simulink model "VL29"  (Simulink 10.1)
settings: Solver=ode3  StartTime=0.0  StopTime=10000.0  FixedStep=Auto  RelTol=1e-3  EnableMultiTasking=on
values from neighbouring files (symbols this model uses):
  In1 = 1    [juece.m]
  In2 = 1    [juece.m]
undefined symbols (not defined in the file): kd1, kd2, ki1, ki2, kp1, kp2
settings Model: Creator=l  LastModifiedBy=97038
settings SolverCC: ShapePreserveControl=EnableAll
settings DataIOCC: LimitDataPoints=on
settings DebuggingCC: UnderspecifiedInitializationDetection=Simplified  MergeDetectMultiDrivingBlocksExec=error  SolverPrmCheckMsg=warning  SFExecutionAtInitializationDiag=warning
settings GRTTargetCC: CombineOutputUpdateFcns=on  GRTInterface=off
settings ConfigComp: CovSFcnEnable=off

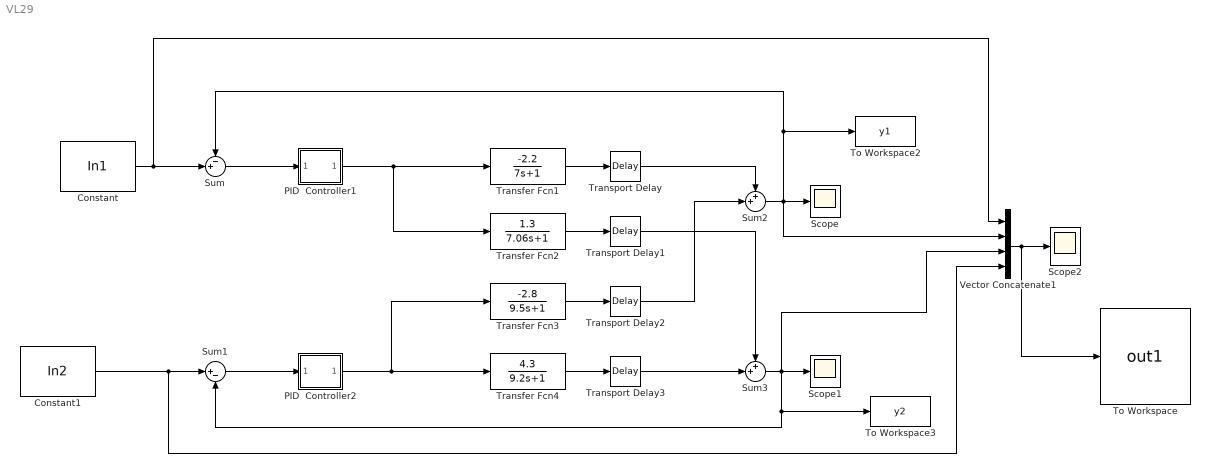
== system VL29 ==
  Constant : Constant  Value=In1
  Constant1 : Constant  Value=In2
  PID  Controller1 : Subsystem  mask(PID Controller){P=kp1, I=ki1, D=kd1}
      mask prompts: P "Proportional:"; I "Integral"; D "Derivative:"
      mask help:
      | Enter expressions for proportional, integral, and derivative terms.
      | P+I/s+Ds
      mask Help: This block implements a PID controller where parameters are entered for the Proportional, Integral and Derivative terms. Unmask this block to see how it works. The derivative term is implemented using a true derivative block.
      mask Display: disp('PID')
  PID  Controller2 : Subsystem  mask(PID Controller){P=kp2, I=ki2, D=kd2}
      mask prompts: P "Proportional:"; I "Integral"; D "Derivative:"
      mask help:
      | Enter expressions for proportional, integral, and derivative terms.
      | P+I/s+Ds
      mask Help: This block implements a PID controller where parameters are entered for the Proportional, Integral and Derivative terms. Unmask this block to see how it works. The derivative term is implemented using a true derivative block.
      mask Display: disp('PID')
  Scope : Scope
  Scope1 : Scope
  Scope2 : Scope
  Sum : Sum  Inputs=-+|  SampleTime=1
  Sum1 : Sum  Inputs=|+-  SampleTime=1
  Sum2 : Sum  Inputs=++|  SampleTime=1
  Sum3 : Sum  Inputs=++|  SampleTime=1
  To Workspace : ToWorkspace  VariableName=out1  SaveFormat=Timeseries  SampleTime=-1
  To Workspace2 : ToWorkspace  VariableName=y1  SampleTime=-1
      settings: Save2DSignal=2-D array (concatenate along first dimension)
  To Workspace3 : ToWorkspace  VariableName=y2  SampleTime=-1
      settings: Save2DSignal=2-D array (concatenate along first dimension)
  Transfer Fcn1 : TransferFcn  Numerator=[-2.2]  Denominator=[7 1]  ContinuousStateAttributes='G11'
  Transfer Fcn2 : TransferFcn  Numerator=[1.3]  Denominator=[7.06 1]  ContinuousStateAttributes='G12'
  Transfer Fcn3 : TransferFcn  Numerator=[-2.8]  Denominator=[9.5 1]
  Transfer Fcn4 : TransferFcn  Numerator=[4.3]  Denominator=[9.2 1]
  Transport Delay : TransportDelay
  Transport Delay1 : TransportDelay  DelayTime=0.3
  Transport Delay2 : TransportDelay  DelayTime=1.8
  Transport Delay3 : TransportDelay  DelayTime=0.35
  Vector Concatenate1 : Concatenate  NumInputs=4
  wires:
  Transfer Fcn1/1 -> Transport Delay/1
  Transfer Fcn2/1 -> Transport Delay1/1
  Transfer Fcn3/1 -> Transport Delay2/1
  Transfer Fcn4/1 -> Transport Delay3/1
  PID  Controller1/1(Out_1) -> Transfer Fcn2/1, Transfer Fcn1/1
  PID  Controller2/1(Out_1) -> Transfer Fcn3/1, Transfer Fcn4/1
  Sum3/1 -> Vector Concatenate1/3, Scope1/1, To Workspace3/1, Sum1/2
  Sum/1 -> PID  Controller1/1(In_1)
  Sum1/1 -> PID  Controller2/1(In_1)
  Constant1/1 -> Vector Concatenate1/4, Sum1/1
  Transport Delay/1 -> Sum2/1
  Transport Delay3/1 -> Sum3/2
  Sum2/1 -> Vector Concatenate1/2, To Workspace2/1, Sum/1, Scope/1
  Vector Concatenate1/1 -> To Workspace/1, Scope2/1
  Transport Delay1/1 -> Sum3/1
  Transport Delay2/1 -> Sum2/2
  Constant/1 -> Vector Concatenate1/1, Sum/2

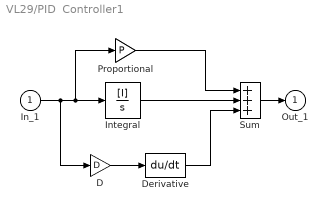
== system VL29/PID  Controller1 ==
  In_1 : Inport
  D : Gain  Gain=D  SaturateOnIntegerOverflow=on  OutDataTypeStr=Inherit: Same as input  ParamDataTypeStr=Inherit: Same as input
  Derivative : Derivative
  Integral : TransferFcn  Numerator=[I]  Denominator=[1 0]
  Proportional : Gain  Gain=P  SaturateOnIntegerOverflow=on  OutDataTypeStr=Inherit: Same as input  ParamDataTypeStr=Inherit: Same as input
  Sum : Sum  Inputs=+++  InputSameDT=on  SaturateOnIntegerOverflow=on  OutDataTypeStr=Inherit: Same as first input
  Out_1 : Outport  InitialOutput=0
  wires:
  D/1 -> Derivative/1
  Sum/1 -> Out_1/1
  In_1/1 -> D/1, Proportional/1, Integral/1
  Derivative/1 -> Sum/3
  Integral/1 -> Sum/2
  Proportional/1 -> Sum/1

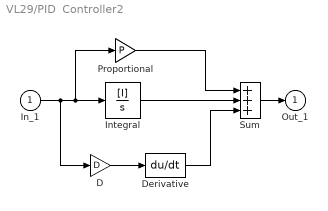
== system VL29/PID  Controller2 ==
  In_1 : Inport
  D : Gain  Gain=D  SaturateOnIntegerOverflow=on  OutDataTypeStr=Inherit: Same as input  ParamDataTypeStr=Inherit: Same as input
  Derivative : Derivative
  Integral : TransferFcn  Numerator=[I]  Denominator=[1 0]
  Proportional : Gain  Gain=P  SaturateOnIntegerOverflow=on  OutDataTypeStr=Inherit: Same as input  ParamDataTypeStr=Inherit: Same as input
  Sum : Sum  Inputs=+++  InputSameDT=on  SaturateOnIntegerOverflow=on  OutDataTypeStr=Inherit: Same as first input
  Out_1 : Outport  InitialOutput=0
  wires:
  D/1 -> Derivative/1
  Sum/1 -> Out_1/1
  In_1/1 -> D/1, Proportional/1, Integral/1
  Derivative/1 -> Sum/3
  Integral/1 -> Sum/2
  Proportional/1 -> Sum/1
